simulink library "flatball_6dof_plnt_lib"  (R2021b)
settings: Solver=VariableStepAuto  StartTime=0.0  StopTime=10.0  RelTol=1e-3
values from neighbouring files (symbols this model uses):
  amb = evalin( 'base', 'amb')    [flatball_6dof_eqom.m]
  C = evalin( 'base', 'C')    [flatball_6dof_eqom.m]
  disc = evalin( 'base', 'disc')    [flatball_6dof_eqom.m]    (also in flatball_6dof_init.m = struct; flatball_init_disc_params.m = struct)
  X0_z1m_at_rest = [1e-3 1e-3 -1, -1e-6 1e-6 -1e-6, 0 0 1e-6, 0 0 -1e-6]    [flatball_6dof_wrk.m]    (also in hummel_thesis_mdl_validation.m)
  Y0 = [0 0 -1, 0 15*C.DEG2RAD 0, 15 0 0, 0 0 (2*15*0.29/disc.d)]    [flatball_6dof_eqom.m]
undefined symbols (not defined in the file or in its folder): CandP, flatball
libraries: simulink x6, aerolibanim x2, aerolibnav x2, matrix_library x2, $bdroot x1, mspfiltlib x1
(part 3 of 3)

== matlab function flatball_6dof_plnt_lib/flatball-6dof-HandH/calc-F-M/lab/calc-F/q-inf/X-to-vel ==
  data: X input; vel output
function vel = fcn( X)
xdot = X(4); ydot = X(5); zdot = X(6);
vel = [xdot ydot zdot];

== matlab function flatball_6dof_plnt_lib/flatball-6dof-HandH/calc-F-M/lab/calc-F/X-to-vel ==
  data: X input; vel output
function vel = fcn( X)
xdot = X(4); ydot = X(5); zdot = X(6);
vel = [xdot ydot zdot];

== matlab function flatball_6dof_plnt_lib/flatball-6dof-HandH/calc-F-M/lab/calc-M/X-to-vel ==
  data: X input; vel output
function vel = fcn( X)
xdot = X(4); ydot = X(5); zdot = X(6);
vel = [xdot ydot zdot];

== matlab function flatball_6dof_plnt_lib/flatball-6dof-HandH/calc-F-M/lab/calc-F/calc-F ==
  data: vel input; F output; T_c_N input; Fg_N input; CLift input; CDrag input; q_inf_times_S input
function F = fcn( vel, T_c_N, Fg_N, CLift, CDrag, q_inf_times_S)
%%
T_c_Npsi = T_c_N(3,:);

vc3 = dot( vel, T_c_Npsi);
v_N = [ vel - vc3*T_c_Npsi];
vmag = norm( vel);
uvel = vel / vmag;
uv_N = v_N / norm( v_N);
u_lat = cross( T_c_Npsi, uv_N);

lift = CLift * q_inf_times_S;
ulift = -cross( uvel, u_lat);

drag = CDrag * q_inf_times_S;
udrag = -uvel;

Faero = lift*ulift + drag*udrag;

F = Faero' + Fg_N;

== matlab function flatball_6dof_plnt_lib/flatball-6dof-HandH/calc-F-M/lab/calc-M/calc-M ==
  data: vel input; M output; T_c_N input; wD_N_inN input; CMpitch input; q_inf_times_Sd input
function M = fcn( vel, T_c_N, wD_N_inN, CMpitch, q_inf_times_Sd)
%% define ambient parameters
amb.g = 9.81; % m/s^2
amb.rho = 1.23; % Kg/m^3

%% define non-aerodynamic parameters
disc = struct;
disc.m = 0.175; % Kg
disc.A = 0.057; % m^2
disc.d = 2*sqrt(0.057/pi); % 2*sqrt(disc.A/pi); % diameter
disc.Ia = 0.002352; % moment of inertia about the spinning axis
disc.Id = 0.001219; % moment of inertia about the planar axis'

%% crowther and potts - per hummel and hubbard
disc.CMq= -1.44e-2;
disc.CNr = -7.1e-6; % short flights
% disc.CNr = -3.41e-5; % long flight f2302
disc.CRr = 3e-3; % NOTE: missing from 2014, borrowed from P&C
disc.CRp =-5.5e-3; % NOTE: missing from 2014, borrowed from P&C
% disc.CLr = 0.0004;
% disc.CLp = -0.013;
% 

%% helper variables
T_c_Npsi = T_c_N(3,:);

%% aerodynamic forces and moments in N reference frame
vc3 = dot( vel, T_c_Npsi);
v_N = [ vel - vc3*T_c_Npsi];

uv_N = v_N / norm( v_N);
u_lat = cross( T_c_Npsi, uv_N);

w_v_N = dot( wD_N_inN, uv_N);
q = dot( wD_N_inN, u_lat);
r = dot( wD_N_inN, T_c_Npsi);
%%
Mv_N = q_inf_times_Sd * (sqrt(disc.d/amb.g)*disc.CRr*r + disc.CRp*w_v_N) * uv_N;
Mpitch = q_inf_times_Sd * (CMpitch + disc.CMq * q) * u_lat;
Mspin = [0 0 disc.CNr*r];
M = T_c_N*Mv_N' + T_c_N*Mpitch' + Mspin';

== matlab function flatball_6dof_plnt_lib/flatball-6dof-HandH/calc-F-M/lab/wrk/flatball_6dof_v1p0 ==
  data: X input; Xdot output; lift output; drag output; alpha output; AdvR output; E_trans output; E_rot output
function [Xdot, lift, drag, alpha, AdvR, E_trans, E_rot]  = flatball_6dof_eom( X)
% flatball equations of motion - NED (north-east-down) configuration
%

%% internal states
x = X(1); y = X(2); z = X(3);
xdot = X(4); ydot = X(5); zdot = X(6);

phi = X(7); theta = X(8); gamma = X(9);
phidot = X(10); thetadot = X(11); gammadot = X(12);

Xdot = zeros(1,12);

%% define ambient parameters
amb.g = 9.81; % m/s^2
amb.rho = 1.23; % Kg/m^3

%% define non-aerodynamic parameters
disc = struct;
disc.m = 0.175; % Kg
disc.A = 0.057; % m^2
disc.d = 2*sqrt(0.057/pi); % 2*sqrt(disc.A/pi); % diameter
disc.Ia = 0.002352; % moment of inertia about the spinning axis
disc.Id = 0.001219; % moment of inertia about the planar axis'

disc.alpha0 = -0.052; %-4 * pi/180.0;

%% THE THREE ESTIMATED COEFFICIENTS
disc.CMq= -1.44E-02;
disc.CRp =-1.25E-02;
disc.CNr = -3.41E-05; % long flight f2302

%% THE seven COEFFICIENTS estimated from three flights
disc.CL0= 0.13; %c&p 07
disc.CLa= 3.09; %c&p 07
disc.CD0= 0.085; %c&p 07
disc.CDa= 3.30; %c&p 07
disc.CM0= -0.01; %c&p 07
disc.CMa= 0.057; %c&p 07 
disc.CRr= 0.00171; % for nondimensionalization = sqrt(d/g), magnitude of CRr changes

%% CL =[ rad CL deg]
disc.CL_data=[ -0.1745 -0.2250 -10; ...
-0.05236 0 -3; ...
0 0.150 0; ...
0.08727 0.4500 5; ...
0.17453 0.7250 10; ...
0.26180 0.9750 15; ...
0.34907 1.2000 20; ...
0.43633 1.4500 25; ...
0.52360 1.6750 30];

%% CD =[ rad CD deg]
disc.CD_data=[ -0.1745 0.1500 -10; ...
-0.05236 0.0800 -3; ...
0 0.1000 0; ...
0.08727 0.1500 5; ...
0.1745 0.2600 10; ...
0.26180 0.3900 15; ...
0.3491 0.5700 20; ...
0.4363 0.7500 25; ...
0.5236 0.9200 30];

%% CM =[ rad CM deg]
disc.CM_data=[-0.174532925 -0.0380 -10; ...
-0.087266463 -0.0220 -5; ...
-0.052359878 -0.0140 -3; ...
0 -0.0060 0; ...
0.052359878 -0.0060 3; ...
0.104719755 -0.0020 6; ...
0.157079633 0.0000 9; ...
0.20943951 0.0100 12; ...
0.261799388 0.0220 15; ...
0.34906585 0.0440 20; ...
0.401425728 0.0600 23; ...
0.453785606 0.0840 26; ...
0.523598776 0.1100 30];

%% helper variables
sin_theta = sin( theta);
cos_theta = cos( theta);
sin_phi = sin( phi);
cos_phi = cos(phi);

% c = T_c_N * N --> transformation matrix T_c_N in N reference frame
T_c_N = [cos_theta sin_theta*sin_phi -sin_theta*cos_phi;
    0 cos_phi sin_phi;
    sin_theta -cos_theta*sin_phi cos_theta*cos_phi];
% c1 = T_c_N(1,:);
% c2 = T_c_N(2,:);
c3 = T_c_N(3,:);

%% aerodynamic forces and moments in N reference frame
vel = [xdot ydot zdot];
vmag = norm( vel);
vc3 = dot( vel, c3);
v_N = [ vel - vc3*c3];
Adp = 0.5 * disc.A * amb.rho * vmag*vmag;
uvel = vel / vmag;
uv_N = v_N / norm( v_N);
u_lat = cross( c3, uv_N);

wD_N_inC = [phidot*cos_theta thetadot phidot*sin_theta+gammadot];
wD_N_inN = T_c_N' * wD_N_inC';

w_v_N = dot( wD_N_inN, uv_N);
w_lat = dot( wD_N_inN, u_lat);
w_spin = dot( wD_N_inN, c3);

alpha = atan( vc3 / norm( v_N)); % angle of attack
AdvR = disc.d * w_spin / 2 / vmag; % advance ratio
E_trans = 0.5 * disc.m * vmag*vmag; % translational energy
E_rot = 0.5 * disc.Ia * gammadot*gammadot; % rotational energy

%% hacks
k_spin_down_decay = 0.25;
% k_CL_gain = 1.0; %2.5;
% k_CD_gain = 1.0; %1.5;
% k_M_gain = 1.0;

%% coefficients - f(alpha)
dalpha = alpha - disc.alpha0;
CL = disc.CL0 + disc.CLa * alpha;
CD = disc.CD0 + disc.CDa * dalpha*dalpha;
CM = disc.CM0 + disc.CMa * alpha;
Mv_N = Adp * disc.d * (sqrt(disc.d/amb.g)*disc.CRr*w_spin + disc.CRp*w_v_N) * uv_N;

%% coefficients - lookup based
% 
% CL = interp1( disc.CL_data(:,1), disc.CL_data(:,2).*k_CL_gain, alpha, 'spline');
% CD = interp1( disc.CD_data(:,1), disc.CD_data(:,2).*k_CD_gain, alpha, 'spline');
% CM = interp1( disc.CM_data(:,1), disc.CM_data(:,2).*k_M_gain, alpha, 'spline');
% % CRr = interp2( disc.CRr_rad, disc.CRr_AdvR, disc.CRr_data, alpha, AdvR,'spline');
% Mv_N = Adp * disc.d * ( disc.CRr* + disc.CRp*w_v_N) * uv_N;

%%
lift = CL * Adp;
drag = CD * Adp;
ulift = -cross( uvel, u_lat);
udrag = -uvel;
Faero = lift*ulift + drag*udrag;
Fg_N = [0 0 disc.m*amb.g]';

F = Faero' + Fg_N;

Mlat = Adp * disc.d * (CM + disc.CMq * w_lat) * u_lat;
Mspin = [0 0 disc.CNr*w_spin];
M = T_c_N * Mv_N' + T_c_N*Mlat' + Mspin';

%%
xdotdot = F(1) / disc.m;
ydotdot = F(2) / disc.m;
zdotdot = F(3) / disc.m;

phidotdot = (M(1) + disc.Id*thetadot*phidot*sin_theta - disc.Ia*thetadot*(phidot*sin_theta+gammadot) + disc.Id*thetadot*phidot*sin_theta)/disc.Id/cos_theta; 
thetadotdot = (M(2) + disc.Ia*phidot*cos_theta*(phidot*sin_theta +gammadot) - disc.Id*phidot*phidot*cos_theta*sin_theta)/disc.Id;
gammadotdot = (M(3) - disc.Ia*(k_spin_down_decay*gammadot*sin_theta + thetadot*phidot*cos_theta))/disc.Ia;

% bug in hummels report?
% gammadotdot = (M(3) - disc.Ia*(phidotdot*sin_theta + thetadot*phidot*cos_theta))/disc.Ia;
% bug in hummels report?
% w/phidotdot term, there is no decay in gammadot
% w/out gammadot term - there is no decay in gammadot
% NOTE: w/it, the decay is too agressive
% FIXME: investigate why this term is necessary for more appropriate
% spindown (based on my data)

%%
Xdot(1) = xdot;
Xdot(2) = ydot;
Xdot(3) = zdot;

Xdot(4) = xdotdot;
Xdot(5) = ydotdot;
Xdot(6) = zdotdot;

Xdot(7) = phidot;
Xdot(8) = thetadot;
Xdot(9) = gammadot;

Xdot(10) = phidotdot;
Xdot(11) = thetadotdot;
Xdot(12) = gammadotdot;

== matlab function flatball_6dof_plnt_lib/flatball-6dof-HandH/calc-F-M/lab/calc-M/q-inf/X-to-vel ==
  data: X input; vel output
function vel = fcn( X)
xdot = X(4); ydot = X(5); zdot = X(6);
vel = [xdot ydot zdot];

== matlab function flatball_6dof_plnt_lib/flatball-6dof-HandH/calc-F-M/lab/calc-M/q-inf/vector-norm ==
  data: vec input; norm output
function norm = fcn( vec)

norm = sqrt( vec(1)*vec(1) + vec(2)*vec(2) + vec(3)*vec(3));

== matlab function flatball_6dof_plnt_lib/flatball-6dof-HandH/calc-F-M/lab/internals ==
  data: X input; AdvR output; E_trans output; E_rot output; T_c_N input; wD_N_inN input
function [ AdvR, E_trans, E_rot]  = internals( X, T_c_N, wD_N_inN)
%% internal states
x = X(1); y = X(2); z = X(3);
xdot = X(4); ydot = X(5); zdot = X(6);

phi = X(7); theta = X(8); gamma = X(9);
phidot = X(10); thetadot = X(11); gammadot = X(12);

%% define non-aerodynamic parameters
disc = struct;
disc.m = 0.175; % Kg
disc.A = 0.057; % m^2
disc.d = 2*sqrt(0.057/pi); % 2*sqrt(disc.A/pi); % diameter
disc.Ia = 0.002352; % moment of inertia about the spinning axis
disc.Id = 0.001219; % moment of inertia about the planar axis'

%% helper variables
vel = [xdot ydot zdot];

T_c_Npsi = T_c_N(3,:);

vmag = norm( vel);

r = dot( wD_N_inN, T_c_Npsi);

AdvR = disc.d * r / 2 / vmag; % advance ratio
E_trans = 0.5 * disc.m * vmag*vmag; % translational energy
E_rot = 0.5 * disc.Ia * gammadot*gammadot; % rotational energy

== matlab function flatball_6dof_plnt_lib/flatball-6dof-HandH/earth-accelerations/calc-THdot ==
  data: X input; M input; dTHdt2 output
function dTHdt2   = f_rot( X, M)
% flatball equations of motion - NED (north-east-down) configuration
%

%% internal states
phi = X(4); theta = X(5); gamma = X(6);
p = X(10); q = X(11); r = X(12);

dTHdt2 = zeros(3,1);

%% define non-aerodynamic parameters
disc = struct;
disc.Ia = 0.002352; % moment of inertia about the spinning axis
disc.Id = 0.001219; % moment of inertia about the planar axis'

%% add in external forces and moments here
phidotdot = (M(1) + disc.Id*q*p*sin(theta) - disc.Ia*q*(p*sin(theta)+r) + disc.Id*q*p*sin(theta))/disc.Id/cos(theta); 
thetadotdot = (M(2) + disc.Ia*p*cos(theta)*(p*sin(theta) +r) - disc.Id*p*p*cos(theta)*sin(theta))/disc.Id;
gammadotdot = (M(3) - disc.Ia*(r*sin(theta) + q*p*cos(theta)))/disc.Ia;

% bug in hummels report?
% gammadotdot = (M(3) - disc.Ia*(phidotdot*sin(theta) + thetadot*phidot*cos(theta)))/disc.Ia;
% bug in hummels report?
% w/phidotdot term, there is no decay in gammadot
% w/out gammadot term - there is no decay in gammadot
% NOTE: w/it, the decay is too agressive
% FIXME: investigate why this term is necessary for more appropriate
% spindown (based on my data)

%%
% dTHdt2(1) = p;
% dTHdt2(2) = q;
% dTHdt2(3) = r;

dTHdt2(1) = phidotdot;
dTHdt2(2) = thetadotdot;
dTHdt2(3) = gammadotdot;

== matlab function flatball_6dof_plnt_lib/flatball-6dof-HandH/calc-F-M/calc-alpha/calc-alpha ==
  data: dXdt input; alpha output; T_c_N input
function alpha  = f( dXdt, T_c_N)
%% internal states
u = dXdt(1); v = dXdt(2); w = dXdt(3);

%% helper variables
T_c_Npsi = T_c_N(3,:);

vel = [u v w];
vc3 = dot( vel, T_c_Npsi);
v_N = vel - vc3*T_c_Npsi;

alpha = atan( vc3 / norm( v_N)); % angle of attack

== matlab function flatball_6dof_plnt_lib/flatball-6dof-HandH/Subsystem/attitude-transform ==
  data: T output; TH input
function T = Ta( TH)
% attitude transformation per Etkin and Reid 1995
phi = TH(1); theta = TH(2); psi = TH(3);
T = [
    cos(theta)*cos(psi), sin(phi)*sin(theta)*cos(psi) - cos(phi)*sin(psi), cos(phi)*sin(theta)*cos(psi) + sin(phi)*sin(psi);
    cos(theta)*sin(psi), sin(phi)*sin(theta)*sin(psi) + cos(phi)*cos(psi), cos(phi)*sin(theta)*sin(psi) - sin(phi)*cos(psi);
    -sin(theta), sin(phi)*cos(theta), cos(phi)*cos(theta)
    ];

== matlab function flatball_6dof_plnt_lib/flatball-6dof-HandH/calc-F-M/calc-F/calc-F ==
  data: vel input; F output; T_c_N input; Fg_N input; CLift input; CDrag input; q_inf_times_S input; lift output; drag output; vmag output
function [F, lift, drag, vmag] = fcn( vel, T_c_N, Fg_N, CLift, CDrag, q_inf_times_S)
%%
T_c_Npsi = T_c_N(3,:);

vc3 = dot( vel', T_c_Npsi);
v_N = vel' - vc3*T_c_Npsi;
vmag = norm( vel');
uvel = vel' / vmag;
uv_N = v_N / norm( v_N);
u_lat = cross( T_c_Npsi, uv_N);

lift = CLift * q_inf_times_S;
ulift = -cross( uvel, u_lat);

drag = CDrag * q_inf_times_S;
udrag = -uvel;

Faero = lift*ulift + drag*udrag;

F = Faero' + Fg_N;

== matlab function flatball_6dof_plnt_lib/flatball-6dof-HandH/Subsystem/rate-transform ==
  data: T output; TH input
function T = Tr( TH)
% euler angle rate transformation per Etkin and Reid 1995
phi = TH(1); theta = TH(2); % psi = TH(3);
T = [
    1, sin(phi)*tan(theta), cos(phi)*tan(theta);
    0, cos(phi), -sin(phi);
    0, sin(phi)*sec(theta), cos(phi)*sec(theta)
    ];

== matlab function flatball_6dof_plnt_lib/flatball-6dof-HandH/calc-F-M/calc-F/q-inf/vector-norm ==
  data: vec input; norm output
function norm = fcn( vec)

norm = sqrt( vec(1)*vec(1) + vec(2)*vec(2) + vec(3)*vec(3));

== matlab function flatball_6dof_plnt_lib/flatball-6dof-HandH/calc-Xdot1/calc-THdot ==
  data: X input; M input; dTHdt2 output; Mlaunch input
function dTHdt2   = f_rot( X, M, Mlaunch)
% flatball equations of motion - NED (north-east-down) configuration
%

%% internal states
phi = X(4); theta = X(5); gamma = X(6);
p = X(10); q = X(11); r = X(12);

dTHdt2 = zeros(3,1);

%% define non-aerodynamic parameters
disc = struct;
disc.Ia = 0.002352; % moment of inertia about the spinning axis
disc.Id = 0.001219; % moment of inertia about the planar axis'

%% add in external forces and moments here
phidotdot = ((M(1) + Mlaunch(1)) + disc.Id*q*p*sin(theta) - disc.Ia*q*(p*sin(theta)+r) + disc.Id*q*p*sin(theta))/disc.Id/cos(theta); 
thetadotdot = ((M(2) + Mlaunch(2)) + disc.Ia*p*cos(theta)*(p*sin(theta) +r) - disc.Id*p*p*cos(theta)*sin(theta))/disc.Id;
gammadotdot = ((M(3) + Mlaunch(3)) - disc.Ia*(r*sin(theta) + q*p*cos(theta)))/disc.Ia;

% bug in hummels report?
% gammadotdot = (M(3) - disc.Ia*(phidotdot*sin(theta) + thetadot*phidot*cos(theta)))/disc.Ia;
% bug in hummels report?
% w/phidotdot term, there is no decay in gammadot
% w/out gammadot term - there is no decay in gammadot
% NOTE: w/it, the decay is too agressive
% FIXME: investigate why this term is necessary for more appropriate
% spindown (based on my data)

%%
% dTHdt2(1) = p;
% dTHdt2(2) = q;
% dTHdt2(3) = r;

dTHdt2(1) = phidotdot;
dTHdt2(2) = thetadotdot;
dTHdt2(3) = gammadotdot;

== matlab function flatball_6dof_plnt_lib/flatball-6dof-HandH/calc-F-M/calc-M/calc-M ==
  data: vel input; M output; T_c_N input; wD_N_inN input; q_inf_times_Sd input; CMpitch input; p output; q output; r output
function [M, p, q, r] = fcn( vel, T_c_N, wD_N_inN, q_inf_times_Sd, CMpitch)
%% define ambient parameters
amb.g = 9.81; % m/s^2
amb.rho = 1.23; % Kg/m^3

%% define non-aerodynamic parameters
disc = struct;
disc.m = 0.175; % Kg
disc.A = 0.057; % m^2
disc.d = 2*sqrt(0.057/pi); % 2*sqrt(disc.A/pi); % diameter
disc.Ia = 0.002352; % moment of inertia about the spinning axis
disc.Id = 0.001219; % moment of inertia about the planar axis'

%% best fit coefficients - copied to/from init script!
disc.CNr = -3e-5;
disc.CMq= -1e-3;
disc.CRr = 5e-4;
disc.CRp = -1e-2;

%% helper variables
T_c_Npsi = T_c_N(3,:);

vc3 = dot( vel', T_c_Npsi);
v_N = vel' - vc3*T_c_Npsi;

uv_N = v_N / norm( v_N);
u_lat = cross( T_c_Npsi, uv_N);

p = dot( wD_N_inN, uv_N);
q = dot( wD_N_inN, u_lat);
r = dot( wD_N_inN, T_c_Npsi);

%% aerodynamic forces and moments in N reference frame
% - is this original and if so, wtf is the sqrt() business about?
% Mv_N = q_inf_times_Sd * (sqrt(disc.d/amb.g)*disc.CRr*r + disc.CRp*p) * uv_N;
% Mpitch = q_inf_times_Sd * (CMpitch + disc.CMq * q) * u_lat;
% Mspin = [0 0 1] .* disc.CNr*r * q_inf_times_Sd;
% M = T_c_N*Mv_N' + T_c_N*Mpitch' + Mspin';

%% aerodynamic forces and moments in N reference frame
M_roll = q_inf_times_Sd * (disc.CRr*r + disc.CRp*p) * uv_N;
M_pitch = q_inf_times_Sd * (CMpitch + disc.CMq*q) * u_lat;
M_yaw = [0 0 1] .* (q_inf_times_Sd * disc.CNr * r);
M = T_c_N*M_roll' + T_c_N*M_pitch' + M_yaw';

== matlab function flatball_6dof_plnt_lib/flatball-6dof-HandH/calc-Xdot1/calc-Xdot ==
  data: dXdt input; F input; Xdot output; Flaunch input
function Xdot   = f_lin( dXdt, F, Flaunch)
% flatball equations of motion - NED (north-east-down) configuration
%

%% internal states
% x = X(1); y = X(2); z = X(3);
u = dXdt(1); v = dXdt(2); w = dXdt(3);

Xdot = zeros(3,1);

%% define non-aerodynamic parameters
disc = struct;
disc.m = 0.175; % Kg

%%
    xdotdot = (F(1) + Flaunch(1)) / disc.m;
    ydotdot = (F(2) + Flaunch(2)) / disc.m;
    zdotdot = (F(3) + Flaunch(3)) / disc.m;

%%
% Xdot(1) = u;
% Xdot(2) = v;
% Xdot(3) = w;

Xdot(1) = xdotdot;
Xdot(2) = ydotdot;
Xdot(3) = zdotdot;

== matlab function flatball_6dof_plnt_lib/flatball-6dof-HandH/calc-F-M/calc-M/q-inf/vector-norm ==
  data: vec input; norm output
function norm = fcn( vec)

norm = sqrt( vec(1)*vec(1) + vec(2)*vec(2) + vec(3)*vec(3));

== matlab function flatball_6dof_plnt_lib/flatball-6dof-HandH/calc-F-M/T_c_N ==
  data: TH input; T_c_N output
function T_c_N  = f( TH)
%% internal states
phi = TH(1); theta = TH(2);

T_c_N = [
    cos(theta) sin(theta)*sin(phi) -sin(theta)*cos(phi);
    0 cos(phi) sin(phi);
    sin(theta) -cos(theta)*sin(phi) cos(theta)*cos(phi)
    ];

== matlab function flatball_6dof_plnt_lib/flatball-6dof-HandH/calc-F-M/calc-alpha/calc-alpha1 ==
  data: T_c_Npsi output; T_c_N input
function T_c_Npsi  = f( T_c_N)
T_c_Npsi = T_c_N(3,:)';

== matlab function flatball_6dof_plnt_lib/flatball-6dof-HandH/calc-F-M/lab/helpers/Subsystem1/transformation-matrices/Ta ==
  data: TH input; M output
function M  = Ta( TH)
% transformation matrix
%
phi = TH(1); theta = TH(2); psi = TH(3);

cos_theta = cos( theta);
cos_phi = cos( phi);
cos_psi = cos( psi);
sin_phi = sin( phi);
sin_theta = sin( theta);
sin_psi = sin( psi);

M = [ ...
    cos_theta*cos_psi sin_phi*sin_theta*cos_phi-cos_phi*sin_psi cos_phi*sin_theta*cos_psi+sin_phi*sin_psi;
    cos_theta*sin_psi sin_phi*sin_theta*sin_psi+cos_phi*cos_psi cos_phi*sin_theta*sin_psi-sin_phi*cos_psi;
    -sin_theta sin_phi*cos_theta cos_phi*cos_theta
    ];

% tan_theta = tan( theta);
% sec_theta = sec( theta);
% transform_r_phi_thea_psi = [
%     1 sin_phi*tan_theta cos_phi*tan_theta
%     0 cos_phi -sin_phi
%     0 sin_phi*sec_theta cos_phi*sec_theta
%     ];

== matlab function flatball_6dof_plnt_lib/flatball-6dof-CandP/body-accelerations/w-tilde ==
  data: w output; dTH2dt input
function w = w_tilde( dTH2dt)
    p = dTH2dt(1); q = dTH2dt( 2); r = dTH2dt(3);
    w = [0 -r q; r 0 -p; -q p 0];

== matlab function flatball_6dof_plnt_lib/flatball-6dof-HandH/scopes/eml-6dof/aero-coefficients ==
  data: X2dot input; alpha3 output; CX output; CTH output; X3dot input; TH3dot input
function [alpha3, CX, CTH] = flatball_6dof(X2dot, X3dot, TH3dot)
%% define ambient conditions
amb.g = 9.7935; % m/s^2
amb.rho = 1.23; % Kg/m^3
%% define flatball (aka - frisbee)

% non-aerodynamic parameters
disc = struct;
disc.m = 0.175; % Kg
disc.I = [0.001219 0 0; 0 0.001219 0; 0 0 0.002352];
disc.c = 0.275;             % Reference chord length (m)
disc.S = pi*(0.275/2)^2;   % Reference area (m^2)

% define flatball aerodynamic properties
disc.alpha0 = -0.052;
disc.CD0 = 0.085;
disc.CDa = 3.30;
disc.CL0 = 0.13;
disc.CLa = 3.09;
disc.CLp = -1.30;
disc.CM0 = -0.01;
disc.CMa = 0.057;
disc.CMq = -1.40;
disc.CNr = -3e-2;

    % calculate aerodynamic coefficients
    u3 = X3dot(1); w3 = X3dot(3);
    p3 = TH3dot(1); q3 = TH3dot(2); r3 = TH3dot(3);
    v_inf = norm( X2dot);

    alpha3 = atan2( w3, u3);                    % angle of attack
    
    CDrag = Cdrag_fcn( alpha3, disc);
    CSide = Cside_fcn( r3, v_inf);
    CLift = Clift_fcn( alpha3, disc);

    CL = CL_fcn( p3, v_inf, disc);
    CM = CM_fcn( alpha3, q3, v_inf, disc);
    CN = CN_fcn( r3, v_inf, disc);

    CX = [-CDrag CSide -CLift];
    CTH = [CL CM CN];
end

function C = Cdrag_fcn( alpha3, disc)
    C = disc.CD0 + disc.CDa * (alpha3 - disc.alpha0)^2;
end

function C = Clift_fcn( alpha3, disc)
    C = disc.CL0 + disc.CLa * alpha3;
end

function C = Cside_fcn( r3, vinf)
    C = -r3 * vinf * 0;                         % <-- 0 == no side force
end

function C = CL_fcn( p3, vinf, disc)
    C = disc.CLp * p3 * disc.c / (2 * vinf);
end

function C = CM_fcn( alpha, q3, vinf, disc)
    C = disc.CM0 + disc.CMa * alpha;
    C = C + (disc.CMq * q3 * disc.c / (2 * vinf));
end

function C = CN_fcn( r3, vinf, disc)
    C = disc.CNr * r3 * disc.c / (2 * vinf);
end

== matlab function flatball_6dof_plnt_lib/flatball-6dof-HandH/scopes/eml-6dof/body-accelerations ==
  data: X2dotdot output; TH2dotdot output; X2dot input; TH2dot input; F2 input; M2 input
function [X2dotdot, TH2dotdot] = flatball_6dof( X2dot, TH2dot, F2, M2)
%% define flatball (aka - frisbee)

% non-aerodynamic parameters
disc = struct;
disc.m = 0.175; % Kg
disc.I = [0.001219 0 0; 0 0.001219 0; 0 0 0.002352];
disc.c = 0.275;             % Reference chord length (m)
disc.S = pi*(0.275/2)^2;   % Reference area (m^2)

    % calculate body accelerations
    p = TH2dot(1); q = TH2dot( 2); r = TH2dot(3);
    w_tilde = [0 -r q; r 0 -p; -q p 0];
    X2dotdot = (F2 ./ disc.m ) - (w_tilde * X2dot);
    TH2dotdot = disc.I^-1 * (M2 - w_tilde * disc.I * TH2dot);
end

== matlab function flatball_6dof_plnt_lib/flatball-6dof-HandH/scopes/eml-6dof/body-force-and-moments ==
  data: F2 output; M2 output; alpha3 input; beta2 input; Ta12 input; F4 input; M4 input
function [F2, M2] = flatball_6dof( alpha3, beta2, Ta12, F4, M4)
%% define ambient conditions
amb.g = 9.7935; % m/s^2
%% define flatball (aka - frisbee)

% non-aerodynamic parameters
disc = struct;
disc.m = 0.175; % Kg

    % calculate forces and moments
    Ta32 = Ta( [0 0 beta2]);
    Ta34 = Ta( [0 alpha3 0]);
    Ta43 = Ta34';
    
    F2aero = Ta43 * Ta32 * F4;
    mg = (disc.m .* [0 0 amb.g]');
    F2 = F2aero + Ta12 * mg;                    % F2
    M2 = Ta43 * Ta32 * M4;                      % M2
end

function T = Ta( TH) %(phi, theta, psi)
    phi = TH(1); theta = TH(2); psi = TH(3);
    T = [
        cos(theta)*cos(psi), sin(phi)*sin(theta)*cos(psi) - cos(phi)*sin(psi), cos(phi)*sin(theta)*cos(psi) + sin(phi)*sin(psi);
        cos(theta)*sin(psi), sin(phi)*sin(theta)*sin(psi) + cos(phi)*cos(psi), cos(phi)*sin(theta)*sin(psi) - sin(phi)*cos(psi);
        -sin(theta), -sin(phi)*cos(theta), cos(phi)*cos(theta)
        ];
end

== matlab function flatball_6dof_plnt_lib/flatball-6dof-HandH/scopes/eml-6dof/earth-reference ==
  data: X1dot output; TH1dot output; Ta21 output; TH1 input; X2dot input; TH2dot input
function [X1dot, TH1dot, Ta21] = flatball_6dof(TH1, X2dot, TH2dot)
    %phi = TH1(1); theta = TH1(2); psi = TH1(3);
    %TH = [phi theta psi];
    Ta21 = Ta( TH1);
    Tr21 = Tr( TH1);

    X1dot = Ta21 * X2dot;                       % X1-dot
    TH1dot = Tr21 * TH2dot;                     % TH1-dotend
end

function T = Ta( TH) %(phi, theta, psi)
    phi = TH(1); theta = TH(2); psi = TH(3);
    T = [
        cos(theta)*cos(psi), sin(phi)*sin(theta)*cos(psi) - cos(phi)*sin(psi), cos(phi)*sin(theta)*cos(psi) + sin(phi)*sin(psi);
        cos(theta)*sin(psi), sin(phi)*sin(theta)*sin(psi) + cos(phi)*cos(psi), cos(phi)*sin(theta)*sin(psi) - sin(phi)*cos(psi);
        -sin(theta), -sin(phi)*cos(theta), cos(phi)*cos(theta)
        ];
end

function T = Tr( TH) %(phi, theta, psi)
    phi = TH(1); theta = TH(2); % psi = TH(3);
    T = [
        1, sin(phi)*tan(theta), cos(phi)*tan(theta);
        0, cos(phi), -sin(phi);
        0, sin(phi)*sec(theta), cos(phi)*sec(theta)
        ];
end

== matlab function flatball_6dof_plnt_lib/flatball-6dof-HandH/scopes/eml-6dof/side-slip-reference ==
  data: X3dot output; TH3dot output; beta2 output; X2dot input; TH2dot input
function [X3dot, TH3dot, beta2] = flatball_6dof(X2dot, TH2dot)
    % calculate zero sideslip variables
    u2 = X2dot(1); v2 = X2dot(2);
    beta2 = atan2( v2, u2);                     % sideslip angle
    
    Ta32 = Ta( [0 0 beta2]);
    Ta23 = Ta32';

    X3dot = Ta23 * X2dot;                       % X3-dot
    TH3dot = Ta23 * TH2dot;                     % TH3-dot
end

function T = Ta( TH) %(phi, theta, psi)
    phi = TH(1); theta = TH(2); psi = TH(3);
    T = [
        cos(theta)*cos(psi), sin(phi)*sin(theta)*cos(psi) - cos(phi)*sin(psi), cos(phi)*sin(theta)*cos(psi) + sin(phi)*sin(psi);
        cos(theta)*sin(psi), sin(phi)*sin(theta)*sin(psi) + cos(phi)*cos(psi), cos(phi)*sin(theta)*sin(psi) - sin(phi)*cos(psi);
        -sin(theta), -sin(phi)*cos(theta), cos(phi)*cos(theta)
        ];
end

== matlab function flatball_6dof_plnt_lib/flatball-6dof-HandH/scopes/eml-6dof/wind-force-and-moments ==
  data: X2dot input; F4 output; M4 output; CX input; CTH input
function [F4, M4] = flatball_6dof( X2dot, CX, CTH)
%% define ambient conditions
amb.g = 9.7935; % m/s^2
amb.rho = 1.23; % Kg/m^3
%% define flatball (aka - frisbee)

% non-aerodynamic parameters
disc = struct;
disc.m = 0.175; % Kg
disc.I = [0.001219 0 0; 0 0.001219 0; 0 0 0.002352];
disc.c = 0.275;             % Reference chord length (m)
disc.S = pi*(0.275/2)^2;   % Reference area (m^2)

% define flatball aerodynamic properties
disc.alpha0 = -0.052;
disc.CD0 = 0.085;
disc.CDa = 3.30;
disc.CL0 = 0.13;
disc.CLa = 3.09;
disc.CLp = -1.30;
disc.CM0 = -0.01;
disc.CMa = 0.057;
disc.CMq = -1.40;
disc.CNr = -3e-2;
    
    % calculate zero sideslip wind variables
    v_inf = norm( X2dot);
    q_inf = (1/2) * amb.rho * v_inf^2;
    qS = q_inf * disc.S;
    qSc = qS * disc.c;
    
    F4 = qS * CX';                              % F4
    M4 = qSc * CTH';                            % M3
end

== matlab function flatball_6dof_plnt_lib/flatball-6dof-HandH/calc-F-M/lab/wrk/flatball_6dof ==
  data: X input; Xdot output; lift output; drag output; alpha output; AdvR output; E_trans output; E_rot output
function [Xdot, lift, drag, alpha, AdvR, E_trans, E_rot]  = flatball_6dof_eom( X)
% flatball equations of motion - NED (north-east-down) configuration
%

%% internal states
x = X(1); y = X(2); z = X(3);
xdot = X(4); ydot = X(5); zdot = X(6);

phi = X(7); theta = X(8); gamma = X(9);
phidot = X(10); thetadot = X(11); gammadot = X(12);

Xdot = zeros(1,12);

%% define ambient parameters
amb.g = 9.81; % m/s^2
amb.rho = 1.23; % Kg/m^3

%% define non-aerodynamic parameters
disc = struct;
disc.m = 0.175; % Kg
disc.A = 0.057; % m^2
disc.d = 2*sqrt(0.057/pi); % 2*sqrt(disc.A/pi); % diameter
disc.Ia = 0.002352; % moment of inertia about the spinning axis
disc.Id = 0.001219; % moment of inertia about the planar axis'

disc.alpha0 = -4 * pi/180.0;

%% THE THREE ESTIMATED COEFFICIENTS
disc.CMq= -1.44E-02;
disc.CRp =-1.25E-02;
disc.CNr = -3.41E-05; % long flight f2302

%% THE seven COEFFICIENTS estimated from three flights
disc.CL0= 0.3331;
disc.CLa= 1.9124;
disc.CD0= 0.1769;
disc.CDa= 0.685;
disc.CM0= -0.0821;
disc.CMa= 0.4338;
disc.CRr= 0.00171; % for nondimensionalization = sqrt(d/g), magnitude of CRr changes

%% CL =[ rad CL deg]
disc.CL_data=[ -0.1745 -0.2250 -10; ...
-0.05236 0 -3; ...
0 0.150 0; ...
0.08727 0.4500 5; ...
0.17453 0.7250 10; ...
0.26180 0.9750 15; ...
0.34907 1.2000 20; ...
0.43633 1.4500 25; ...
0.52360 1.6750 30];

%% CD =[ rad CD deg]
disc.CD_data=[ -0.1745 0.1500 -10; ...
-0.05236 0.0800 -3; ...
0 0.1000 0; ...
0.08727 0.1500 5; ...
0.1745 0.2600 10; ...
0.26180 0.3900 15; ...
0.3491 0.5700 20; ...
0.4363 0.7500 25; ...
0.5236 0.9200 30];

%% CM =[ rad CM deg]
disc.CM_data=[-0.174532925 -0.0380 -10; ...
-0.087266463 -0.0220 -5; ...
-0.052359878 -0.0140 -3; ...
0 -0.0060 0; ...
0.052359878 -0.0060 3; ...
0.104719755 -0.0020 6; ...
0.157079633 0.0000 9; ...
0.20943951 0.0100 12; ...
0.261799388 0.0220 15; ...
0.34906585 0.0440 20; ...
0.401425728 0.0600 23; ...
0.453785606 0.0840 26; ...
0.523598776 0.1100 30];

%% helper variables
cos_theta = cos( theta);
cos_phi = cos( phi);
cos_psi = cos( psi);
sin_phi = sin( phi);
sin_theta = sin( theta);
sin_psi = sin( psi);
tan_theta = tan( theta);
sec_theta = sec( theta);

transform_a_phi_theta_psi = [ ...
    cos_theta*cos_psi sin_phi*sin_theta*cos_phi-cos_phi*sin_psi cos_phi*sin_theta*cos_psi+sin_phi*sin_psi;
    cos_theta*sin_psi sin_phi*sin_theta*sin_psi+cos_phi*cos_psi cos_phi*sin_theta*sin_psi-sin_phi*cos_psi;
    -sin_theta sin_phi*cos_theta cos_phi*cos_theta
    ];
transform_r_phi_thea_psi = [
    1 sin_phi*tan_theta cos_phi*tan_theta
    0 cos_phi -sin_phi
    0 sin_phi*sec_theta cos_phi*sec_theta
    ];
% c1 = T_c_N(1,:);
% c2 = T_c_N(2,:);
c3 = T_c_N(3,:);

%% aerodynamic forces and moments in N reference frame
vel = [xdot ydot zdot];
vmag = norm( vel);
vc3 = dot( vel, c3);
v_N = [ vel - vc3*c3];
Adp = 0.5 * disc.A * amb.rho * vmag*vmag;
uvel = vel / vmag;
uv_N = v_N / norm( v_N);
u_lat = cross( c3, uv_N);

wD_N_inC = [phidot*cos_theta thetadot phidot*sin_theta+gammadot];
wD_N_inN = T_c_N' * wD_N_inC';

w_v_N = dot( wD_N_inN, uv_N);
w_lat = dot( wD_N_inN, u_lat);
w_spin = dot( wD_N_inN, c3);

alpha = atan( vc3 / norm( v_N)); % angle of attack
AdvR = disc.d * w_spin / 2 / vmag; % advance ratio
E_trans = 0.5 * disc.m * vmag*vmag; % translational energy
E_rot = 0.5 * disc.Ia * gammadot*gammadot; % rotational energy

%% coefficients - f(alpha)
% dalpha = alpha - disc.alpha0;
% Cl = disc.CL0 + disc.CLa * alpha;
% CD = disc.CD0 + disc.CDa * dalpha*dalpha;
% CM = disc.CM0 + disc.CMa * alpha;
% Mv_N = Adp * disc.d * (sqrt(disc.d/amb.g)*disc.CRr*w_spin + disc.CRp*w_v_N) * uv_N;

%% coefficients - lookup based
% hacks
k_CL_gain = 1.0; %2.5;
k_CD_gain = 1.0; %1.5;
k_M_gain = 1.0;
k_decay = 0.25;
% hacks

CL = interp1( disc.CL_data(:,1), disc.CL_data(:,2).*k_CL_gain, alpha, 'spline');
CD = interp1( disc.CD_data(:,1), disc.CD_data(:,2).*k_CD_gain, alpha, 'spline');
CM = interp1( disc.CM_data(:,1), disc.CM_data(:,2).*k_M_gain, alpha, 'spline');
% CRr = interp2( disc.CRr_rad, disc.CRr_AdvR, disc.CRr_data, alpha, AdvR,'spline');
Mv_N = Adp * disc.d * ( disc.CRr* + disc.CRp*w_v_N) * uv_N;

%%
lift = CL * Adp;
drag = CD * Adp;
ulift = -cross( uvel, u_lat);
udrag = -uvel;
Faero = lift*ulift + drag*udrag;
Fg_N = [0 0 disc.m*amb.g]';

F = Faero' + Fg_N;

Mlat = Adp * disc.d * (CM + disc.CMq * w_lat) * u_lat;
Mspin = [0 0 disc.CNr*-1e-5*w_spin];
M = T_c_N * Mv_N' + T_c_N*Mlat' + Mspin';

%%
xdotdot = F(1) / disc.m;
ydotdot = F(2) / disc.m;
zdotdot = F(3) / disc.m;

phidotdot = (M(1) + disc.Id*thetadot*phidot*sin_theta - disc.Ia*thetadot*(phidot*sin_theta+gammadot) + disc.Id*thetadot*phidot*sin_theta)/disc.Id/cos_theta; 
thetadotdot = (M(2) + disc.Ia*phidot*cos_theta*(phidot*sin_theta +gammadot) - disc.Id*phidot*phidot*cos_theta*sin_theta)/disc.Id;
% bug in hummels report?
% gammadotdot = (M(3) - disc.Ia*(phidotdot*sin_theta + thetadot*phidot*cos_theta))/disc.Ia;
% bug in hummels report?
% w/phidotdot term, there is no decay in gammadot
% w/out gammadot term - there is no decay in gammadot
% NOTE: w/it, the decay is too agressive
% FIXME: investigate why this term is necessary for more appropriate
% spindown (based on my data)
gammadotdot = (M(3) - disc.Ia*(k_decay*gammadot*sin_theta + thetadot*phidot*cos_theta))/disc.Ia;

%%
Xdot(1) = xdot;
Xdot(2) = ydot;
Xdot(3) = zdot;

Xdot(4) = xdotdot;
Xdot(5) = ydotdot;
Xdot(6) = zdotdot;

Xdot(7) = phidot;
Xdot(8) = thetadot;
Xdot(9) = gammadot;

Xdot(10) = phidotdot;
Xdot(11) = thetadotdot;
Xdot(12) = gammadotdot;

== matlab function flatball_6dof_plnt_lib/flatball-6dof-HandH/scopes/work-in-progress/aero-coefficients/MATLAB Function ==
  data: alpha input; C output
function C = Cdrag( alpha)
    CD0 = 0.085;
    CDa = 3.30;
    alpha0 = -0.052;
    C = CD0 + CDa * (alpha - alpha0)^2;

== matlab function flatball_6dof_plnt_lib/flatball-6dof-HandH/scopes/work-in-progress/aero-coefficients/MATLAB Function2 ==
  data: alpha input; C output
function C = Clift( alpha)
    CL0 = 0.13;
    CLa = 3.09;
    C = CL0 + CLa * alpha;

== matlab function flatball_6dof_plnt_lib/flatball-6dof-HandH/scopes/work-in-progress/aero-coefficients/MATLAB Function3 ==
  data: r3 input; C output; v_inf input
function C = Cside( r3, v_inf)
    C = -r3 * v_inf;

== matlab function flatball_6dof_plnt_lib/flatball-6dof-HandH/scopes/work-in-progress/aero-coefficients/MATLAB Function4 ==
  data: p input; C output; v_inf input; c input
function C = CL( p, v_inf, c)
    CLp = -1.30;
    C = CLp * p * c / (2 * v_inf);

== matlab function flatball_6dof_plnt_lib/flatball-6dof-HandH/scopes/work-in-progress/aero-coefficients/MATLAB Function5 ==
  data: alpha input; C output; q input; v_inf input; c input
function C = CM( alpha, q, v_inf, c)
    CM0 = -0.01;
    CMa = 0.057;
    CMq = -1.40;
    C = CM0 + CMa * alpha;
    C = C + CMq * q * c / (2 * v_inf);

== matlab function flatball_6dof_plnt_lib/flatball-6dof-HandH/scopes/work-in-progress/aero-coefficients/MATLAB Function6 ==
  data: r input; C output; v_inf input; c input
function C = CN( r, v_inf, c)
    CNr = -3e-2;
    C = CNr * r * c / (2 * v_inf);

== matlab function flatball_6dof_plnt_lib/flatball-6dof-HandH/scopes/work-in-progress/body-forces-and-moments/attitude-transformation ==
  data: T output; TH input
function T = Ta( TH) %(phi, theta, psi)
    phi = TH(1); theta = TH(2); psi = TH(3);
    T = [
        cos(theta)*cos(psi), sin(phi)*sin(theta)*cos(psi) - cos(phi)*sin(psi), cos(phi)*sin(theta)*cos(psi) + sin(phi)*sin(psi);
        cos(theta)*sin(psi), sin(phi)*sin(theta)*sin(psi) + cos(phi)*cos(psi), cos(phi)*sin(theta)*sin(psi) - sin(phi)*cos(psi);
        -sin(theta), -sin(phi)*cos(theta), cos(phi)*cos(theta)
        ];
end

== matlab function flatball_6dof_plnt_lib/flatball-6dof-HandH/scopes/work-in-progress/body-forces-and-moments/attitude-transformation1 ==
  data: T output; TH input
function T = Ta( TH) %(phi, theta, psi)
    phi = TH(1); theta = TH(2); psi = TH(3);
    T = [
        cos(theta)*cos(psi), sin(phi)*sin(theta)*cos(psi) - cos(phi)*sin(psi), cos(phi)*sin(theta)*cos(psi) + sin(phi)*sin(psi);
        cos(theta)*sin(psi), sin(phi)*sin(theta)*sin(psi) + cos(phi)*cos(psi), cos(phi)*sin(theta)*sin(psi) - sin(phi)*cos(psi);
        -sin(theta), -sin(phi)*cos(theta), cos(phi)*cos(theta)
        ];
end

== matlab function flatball_6dof_plnt_lib/flatball-6dof-HandH/scopes/work-in-progress/earth-reference/attitude-transformation ==
  data: T output; TH input
function T = Ta( TH) %(phi, theta, psi)
    phi = TH(1); theta = TH(2); psi = TH(3);
    T = [
        cos(theta)*cos(psi), sin(phi)*sin(theta)*cos(psi) - cos(phi)*sin(psi), cos(phi)*sin(theta)*cos(psi) + sin(phi)*sin(psi);
        cos(theta)*sin(psi), sin(phi)*sin(theta)*sin(psi) + cos(phi)*cos(psi), cos(phi)*sin(theta)*sin(psi) - sin(phi)*cos(psi);
        -sin(theta), -sin(phi)*cos(theta), cos(phi)*cos(theta)
        ];
end

== matlab function flatball_6dof_plnt_lib/flatball-6dof-HandH/scopes/work-in-progress/earth-reference/rate-transformation ==
  data: T output; TH input
function T = Tr( TH) %(phi, theta, psi)
    phi = TH(1); theta = TH(2); % psi = TH(3);
    T = [
        1, sin(phi)*tan(theta), cos(phi)*tan(theta);
        0, cos(phi), -sin(phi);
        0, sin(phi)*sec(theta), cos(phi)*sec(theta)
        ];
end

== matlab function flatball_6dof_plnt_lib/flatball-6dof-HandH/scopes/work-in-progress/earth-reference/w_tilde/MATLAB Function ==
  data: X2dot input; w output
function w = w_tilde( X2dot)
    p = X2dot(1); q = X2dot(2); r = X2dot(3);
    w = [
        0 -r q;
        r 0 -p;
        -q p 0
        ];

== matlab function flatball_6dof_plnt_lib/flatball-6dof-HandH/scopes/work-in-progress/eml-6dof/MATLAB Function ==
  data: X1 output; TH1 output; X1dot output; TH1dot output; X2dot output; TH2dot output; X3dot output; TH3dot output; alpha3 output; beta2 output; X input; dydt output; X0 input
function [X1, TH1, X1dot, TH1dot, X2dot, TH2dot, X3dot, TH3dot, alpha3, beta2, dydt] = flatball_6dof(X, X0)
%% define ambient conditions
amb.g = 9.7935; % m/s^2
amb.rho = 1.23; % Kg/m^3
%% define flatball (aka - frisbee)

% non-aerodynamic parameters
disc = struct;
disc.m = 0.175; % Kg
disc.I = [0.001219 0 0; 0 0.001219 0; 0 0 0.002352];
disc.c = 0.275;             % Reference chord length (m)
disc.S = pi*(0.275/2)^2;   % Reference area (m^2)

% define flatball aerodynamic properties
disc.alpha0 = -0.052;
disc.CD0 = 0.085;
disc.CDa = 3.30;
disc.CL0 = 0.13;
disc.CLa = 3.09;
disc.CLp = -1.30;
disc.CM0 = -0.01;
disc.CMa = 0.057;
disc.CMq = -1.40;
disc.CNr = -3e-2;

% NOTE: per simulation of a spin-stabilised sports disc
%       crowther & potts 2007
   
    % unpack state variables
    x = X(1); y = X(2); z = X(3);               % X1
    phi = X(4); theta = X(5); psi = X(6);       % TH1
    u = X(7); v = X(8); w = X(9);               % X2-dot
    p = X(10); q = X(11); r = X(12);            % TH2-dot
  
    % body reference variables
    X2dot = [u v w]';                           % X2-dot
    TH2dot = [p q r]';                          % TH2-dot

    v_inf = norm( X2dot);
    q_inf = (1/2) * amb.rho * v_inf^2;

    % calculate earth reference variables
    X1 = [x y z]';                              % X1
    TH1 = [phi theta psi]';                     % TH1

    Ta21 = Ta( TH1);
    Ta12 = Ta21';
    Tr21 = Tr( TH1);

    X1dot = Ta21 * X2dot;                       % X1-dot
    TH1dot = Tr21 * TH2dot;                     % TH1-dot

    % calculate zero sideslip variables
    u2 = X2dot(1); v2 = X2dot(2);
    beta2 = atan2( v2, u2);                     % sideslip angle
    
    Ta32 = Ta( [0 0 beta2]);
    Ta23 = Ta32';

    X3dot = Ta23 * X2dot;                       % X3-dot
    TH3dot = Ta23 * TH2dot;                     % TH3-dot

    % calculate aerodynamic coefficients
    u3 = X3dot(1); w3 = X3dot(3);
    p3 = TH3dot(1); q3 = TH3dot(2); r3 = TH3dot(3);

    alpha3 = atan2( w3, u3);                    % angle of attack
    
    CDrag = Cdrag_fcn( alpha3, disc);
    CSide = Cside_fcn( r3, v_inf);
    CLift = Clift_fcn( alpha3, disc);

    CL = CL_fcn( p3, v_inf, disc);
    CM = CM_fcn( alpha3, q3, v_inf, disc);
    CN = CN_fcn( r3, v_inf, disc);

    % calculate zero sideslip wind variables
    qS = q_inf * disc.S;
    qSc = qS * disc.c;
    mg = (disc.m .* [0 0 amb.g]');

    % calculate forces and moments
    Ta34 = Ta( [0 alpha3 0]);
    Ta43 = Ta34';
    
    F4 = qS * [-CDrag CSide -CLift]';           % F4
    M4 = qSc * [CL CM CN]';                     % M3

    F2aero = Ta43 * Ta32 * F4;
    F2 = F2aero + Ta12 * mg;                    % F2
    M2 = Ta43 * Ta32 * M4;                      % M2

    % calculate body accelerations
    w_tilde = [0 -r q; r 0 -p; -q p 0];
    X2dotdot = (F2 ./ disc.m ) - (w_tilde * X2dot);
    TH2dotdot = disc.I^-1 * (M2 - w_tilde * disc.I * TH2dot);

    dydt = [X1dot' TH1dot' X2dotdot' TH2dotdot']';
end

function T = Ta( TH) %(phi, theta, psi)
    phi = TH(1); theta = TH(2); psi = TH(3);
    T = [
        cos(theta)*cos(psi), sin(phi)*sin(theta)*cos(psi) - cos(phi)*sin(psi), cos(phi)*sin(theta)*cos(psi) + sin(phi)*sin(psi);
        cos(theta)*sin(psi), sin(phi)*sin(theta)*sin(psi) + cos(phi)*cos(psi), cos(phi)*sin(theta)*sin(psi) - sin(phi)*cos(psi);
        -sin(theta), -sin(phi)*cos(theta), cos(phi)*cos(theta)
        ];
end

function T = Tr( TH) %(phi, theta, psi)
    phi = TH(1); theta = TH(2); % psi = TH(3);
    T = [
        1, sin(phi)*tan(theta), cos(phi)*tan(theta);
        0, cos(phi), -sin(phi);
        0, sin(phi)*sec(theta), cos(phi)*sec(theta)
        ];
end

function C = Cdrag_fcn( alpha3, disc)
    C = disc.CD0 + disc.CDa * (alpha3 - disc.alpha0)^2;
end

function C = Clift_fcn( alpha3, disc)
    C = disc.CL0 + disc.CLa * alpha3;
end

function C = Cside_fcn( r3, vinf)
    C = -r3 * vinf * 0;                         % <-- 0 == no side force
end

function C = CL_fcn( p3, vinf, disc)
    C = disc.CLp * p3 * disc.c / (2 * vinf);
end

function C = CM_fcn( alpha, q3, vinf, disc)
    C = disc.CM0 + disc.CMa * alpha;
    C = C + (disc.CMq * q3 * disc.c / (2 * vinf));
end

function C = CN_fcn( r3, vinf, disc)
    C = disc.CNr * r3 * disc.c / (2 * vinf);
end

== matlab function flatball_6dof_plnt_lib/flatball-6dof-HandH/scopes/work-in-progress/side-slip/attitude-transformation ==
  data: T output; TH input
function T = Ta( TH) %(phi, theta, psi)
    phi = TH(1); theta = TH(2); psi = TH(3);
    T = [
        cos(theta)*cos(psi), sin(phi)*sin(theta)*cos(psi) - cos(phi)*sin(psi), cos(phi)*sin(theta)*cos(psi) + sin(phi)*sin(psi);
        cos(theta)*sin(psi), sin(phi)*sin(theta)*sin(psi) + cos(phi)*cos(psi), cos(phi)*sin(theta)*sin(psi) - sin(phi)*cos(psi);
        -sin(theta), -sin(phi)*cos(theta), cos(phi)*cos(theta)
        ];
end

== matlab function flatball_6dof_plnt_lib/flatball-6dof-CandP/body-forces-and-moments/attitude-transform ==
  data: T output; TH input
function T = Ta( TH)
% attitude transformation per Etkin and Reid 1995
phi = TH(1); theta = TH(2); psi = TH(3);
T = [
    cos(theta)*cos(psi), sin(phi)*sin(theta)*cos(psi) - cos(phi)*sin(psi), cos(phi)*sin(theta)*cos(psi) + sin(phi)*sin(psi);
    cos(theta)*sin(psi), sin(phi)*sin(theta)*sin(psi) + cos(phi)*cos(psi), cos(phi)*sin(theta)*sin(psi) - sin(phi)*cos(psi);
    -sin(theta), sin(phi)*cos(theta), cos(phi)*cos(theta)
    ];

== matlab function flatball_6dof_plnt_lib/flatball-6dof-CandP/earth-reference/attitude-transform ==
  data: T output; TH input
function T = Ta( TH)
% attitude transformation per Etkin and Reid 1995
phi = TH(1); theta = TH(2); psi = TH(3);
T = [
    cos(theta)*cos(psi), sin(phi)*sin(theta)*cos(psi) - cos(phi)*sin(psi), cos(phi)*sin(theta)*cos(psi) + sin(phi)*sin(psi);
    cos(theta)*sin(psi), sin(phi)*sin(theta)*sin(psi) + cos(phi)*cos(psi), cos(phi)*sin(theta)*sin(psi) - sin(phi)*cos(psi);
    -sin(theta), sin(phi)*cos(theta), cos(phi)*cos(theta)
    ];

== matlab function flatball_6dof_plnt_lib/flatball-6dof-HandH/calc-F-M/lab/helpers/Subsystem1/transformation-matrices/Tr ==
  data: TH input; M output
function M  = Tr( TH)
% transformation matrix
%
phi = TH(1); theta = TH(2); psi = TH(3);

cos_theta = cos( theta);
cos_phi = cos( phi);
cos_psi = cos( psi);
sin_phi = sin( phi);
sin_theta = sin( theta);
sin_psi = sin( psi);

tan_theta = tan( theta);
sec_theta = sec( theta);

M = [
    1 sin_phi*tan_theta cos_phi*tan_theta
    0 cos_phi -sin_phi
    0 sin_phi*sec_theta cos_phi*sec_theta
    ];

== matlab function flatball_6dof_plnt_lib/flatball-6dof-CandP/earth-reference/rate-transform ==
  data: T output; TH input
function T = Tr( TH)
% euler angle rate transformation per Etkin and Reid 1995
phi = TH(1); theta = TH(2); % psi = TH(3);
T = [
    1, sin(phi)*tan(theta), cos(phi)*tan(theta);
    0, cos(phi), -sin(phi);
    0, sin(phi)*sec(theta), cos(phi)*sec(theta)
    ];

== matlab function flatball_6dof_plnt_lib/flatball-6dof-CandP/zero-side-slip-reference/attitude-transform ==
  data: T output; TH input
function T = Ta( TH)
% attitude transformation per Etkin and Reid 1995
phi = TH(1); theta = TH(2); psi = TH(3);
T = [
    cos(theta)*cos(psi), sin(phi)*sin(theta)*cos(psi) - cos(phi)*sin(psi), cos(phi)*sin(theta)*cos(psi) + sin(phi)*sin(psi);
    cos(theta)*sin(psi), sin(phi)*sin(theta)*sin(psi) + cos(phi)*cos(psi), cos(phi)*sin(theta)*sin(psi) - sin(phi)*cos(psi);
    -sin(theta), sin(phi)*cos(theta), cos(phi)*cos(theta)
    ];

== matlab function flatball_6dof_plnt_lib/flatball-6dof-HandH/calc-F-M/lab/helpers/Subsystem/Ta1 ==
  data: phi input; T output; theta input; psi input
function T  = Ta( phi, theta, psi)
% transformation matrix
%

cos_theta = cos( theta);
cos_phi = cos( phi);
cos_psi = cos( psi);
sin_phi = sin( phi);
sin_theta = sin( theta);
sin_psi = sin( psi);

T= [ ...
    cos_theta*cos_psi sin_phi*sin_theta*cos_phi-cos_phi*sin_psi cos_phi*sin_theta*cos_psi+sin_phi*sin_psi;
    cos_theta*sin_psi sin_phi*sin_theta*sin_psi+cos_phi*cos_psi cos_phi*sin_theta*sin_psi-sin_phi*cos_psi;
    -sin_theta sin_phi*cos_theta cos_phi*cos_theta
    ];

% tan_theta = tan( theta);
% sec_theta = sec( theta);
% transform_r_phi_thea_psi = [
%     1 sin_phi*tan_theta cos_phi*tan_theta
%     0 cos_phi -sin_phi
%     0 sin_phi*sec_theta cos_phi*sec_theta
%     ];

== matlab function flatball_6dof_plnt_lib/flatball-6dof-HandH/calc-F-M/lab/helpers/Subsystem2/Ta2 ==
  data: phi input; T output; theta input; psi input
function T  = Ta( phi, theta, psi)
% transformation matrix
%

cos_theta = cos( theta);
cos_phi = cos( phi);
cos_psi = cos( psi);
sin_phi = sin( phi);
sin_theta = sin( theta);
sin_psi = sin( psi);

T= [ ...
    cos_theta*cos_psi sin_phi*sin_theta*cos_phi-cos_phi*sin_psi cos_phi*sin_theta*cos_psi+sin_phi*sin_psi;
    cos_theta*sin_psi sin_phi*sin_theta*sin_psi+cos_phi*cos_psi cos_phi*sin_theta*sin_psi-sin_phi*cos_psi;
    -sin_theta sin_phi*cos_theta cos_phi*cos_theta
    ];

% tan_theta = tan( theta);
% sec_theta = sec( theta);
% transform_r_phi_thea_psi = [
%     1 sin_phi*tan_theta cos_phi*tan_theta
%     0 cos_phi -sin_phi
%     0 sin_phi*sec_theta cos_phi*sec_theta
%     ];

== matlab function flatball_6dof_plnt_lib/flatball-6dof-HandH/calc-F-M/lab/helpers/Subsystem1/w_ ==
  data: THdot input; M output
function M  = w_( THdot)
% transformation matrix
%
p = THdot(1); q = THdot(2); r = THdot(3);

M = [ ...
    0 -r q;
    r 0 -p;
    -q p 0
    ];

== matlab function flatball_6dof_plnt_lib/flatball-6dof-HandH/calc-F-M/lab/helpers/Subsystem/zero-side-slip-angle ==
  data: Xdot input; beta output
function beta  = f( Xdot)
% calculate side-slip angle

beta = atan( Xdot(2) / Xdot(1));
